simulink model "with_absorber"  (R2022b)
settings: Solver=VariableStepAuto  StartTime=0.0  StopTime=6  RelTol=1e-6
values from neighbouring files (symbols this model uses):
  c_1 = zeta*2*m1*w_n    (= 14.4568322948)    [A_plus.m]
  F_amp = m*e*w^2    (= 41.1233516712)    [A_plus.m]
  k1 = 38000    [A_plus.m]
  k2 = 17000    [A_plus.m]
  m1 = 0.55    [A_plus.m]
  m2 = 0.125*2    (= 0.25)    [A_plus.m]
  w = 2500*2*pi/60    (= 261.799387799)    [A_plus.m]
settings Model: Creator=a7mad  LastModifiedBy=a7mad

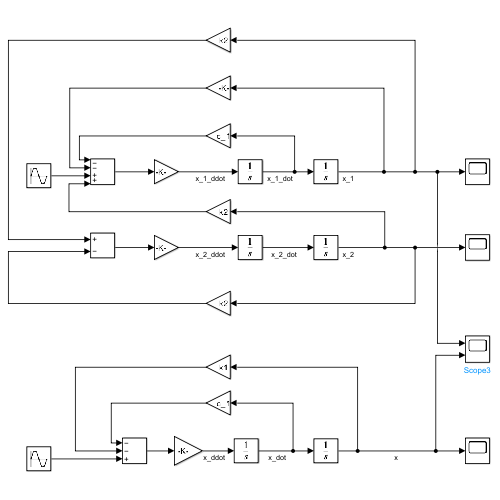
[thumbnail: Simulink's stored preview of the top-level diagram]
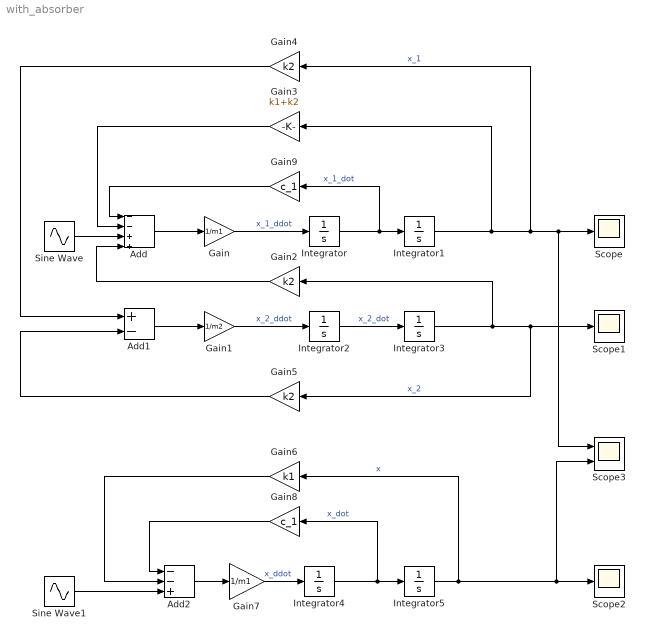
== system with_absorber ==
  Add : Sum  Inputs=--++
  Add1 : Sum  Inputs=+-
  Add2 : Sum  Inputs=--+
  Gain : Gain  Gain=1/m1
  Gain1 : Gain  Gain=1/m2
  Gain2 : Gain  Gain=k2
  Gain3 : Gain  Gain=k1+k2
  Gain4 : Gain  Gain=k2
  Gain5 : Gain  Gain=k2
  Gain6 : Gain  Gain=k1
  Gain7 : Gain  Gain=1/m1
  Gain8 : Gain  Gain=c_1
  Gain9 : Gain  Gain=c_1
  Integrator{,1..5} (6 alike) : Integrator
  Scope : Scope
  Scope1 : Scope
  Scope2 : Scope
  Scope3 : Scope  NumInputPorts=2
  Sine Wave : Sin  Amplitude=F_amp  Frequency=w  SampleTime=0
  Sine Wave1 : Sin  Amplitude=F_amp  Frequency=w  SampleTime=0
  wires:
  Integrator/1 -> Gain9/1, Integrator1/1  "x_1_dot"
  Integrator1/1 -> Gain4/1, Scope3/1, Scope/1, Gain3/1  "x_1"
  Gain/1 -> Integrator/1  "x_1_ddot"
  Integrator3/1 -> Gain2/1, Gain5/1, Scope1/1  "x_2"
  Integrator2/1 -> Integrator3/1  "x_2_dot"
  Gain1/1 -> Integrator2/1  "x_2_ddot"
  Add/1 -> Gain/1
  Add1/1 -> Gain1/1
  Gain5/1 -> Add1/2
  Gain4/1 -> Add1/1
  Integrator5/1 -> Scope3/2, Scope2/1, Gain6/1  "x"
  Add2/1 -> Gain7/1
  Integrator4/1 -> Gain8/1, Integrator5/1  "x_dot"
  Gain7/1 -> Integrator4/1  "x_ddot"
  Gain2/1 -> Add/4
  Sine Wave/1 -> Add/3
  Gain3/1 -> Add/2
  Gain9/1 -> Add/1
  Sine Wave1/1 -> Add2/3
  Gain6/1 -> Add2/2
  Gain8/1 -> Add2/1
